simulink model "B_Inverter1"  (Simulink 8.4)
settings: Solver=ode45  StartTime=0.0  StopTime=1  RelTol=1e-3
libraries: powerlib x10
settings Model: Creator=ELECTRICAL-HOD  LastModifiedBy=INTEL

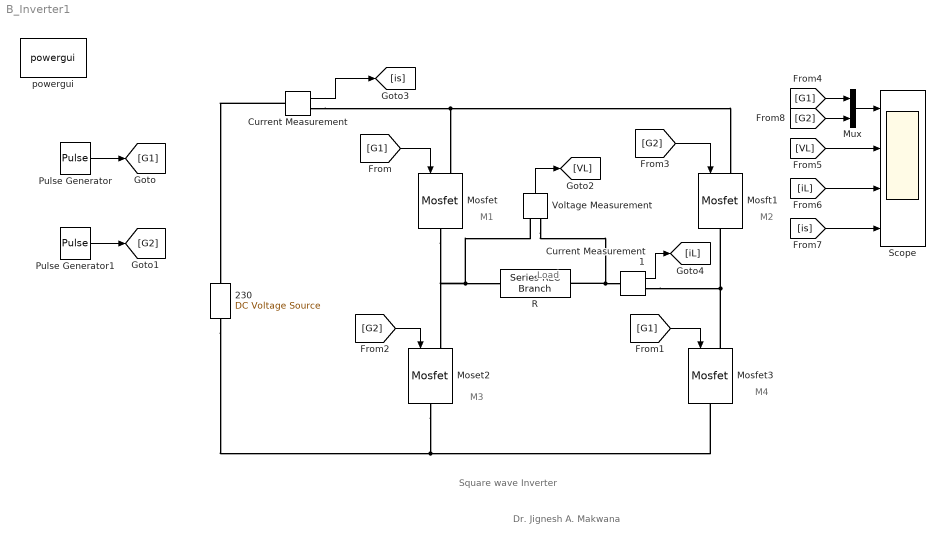
== system B_Inverter1 ==
  note: Load
  note: M1
  note: M4
  note: M3
  note: M2
  note: Dr. Jignesh A. Makwana
  note: Square wave Inverter
  230 : powerlib/Electrical Sources/DC Voltage Source  Amplitude=230  Measurements=None
  Current Measurement : powerlib/Measurements/Current Measurement  PhasorSimulation=off  OutputType=Complex  PSBequivalent=0
  Current Measurement1 : powerlib/Measurements/Current Measurement  PhasorSimulation=off  OutputType=Complex  PSBequivalent=0
  Moset2 : powerlib/Power Electronics/Mosfet  Ron=0.1  Lon=0  Rd=0.01  Vfd=0  IC=0  Rs=1e5  Cs=inf  Measurements=off
  Mosfet : powerlib/Power Electronics/Mosfet  Ron=0.1  Lon=0  Rd=0.01  Vfd=0  IC=0  Rs=1e5  Cs=inf  Measurements=off
  Mosfet3 : powerlib/Power Electronics/Mosfet  Ron=0.1  Lon=0  Rd=0.01  Vfd=0  IC=0  Rs=1e5  Cs=inf  Measurements=off
  Mosft1 : powerlib/Power Electronics/Mosfet  Ron=0.1  Lon=0  Rd=0.01  Vfd=0  IC=0  Rs=1e5  Cs=inf  Measurements=off
  Mux : Mux  Inputs=2
  Pulse Generator : DiscretePulseGenerator  PulseType=Time based  Amplitude=5  Period=0.02  PulseWidth=50
  Pulse Generator1 : DiscretePulseGenerator  PulseType=Time based  Amplitude=5  Period=0.02  PulseWidth=50  PhaseDelay=0.01
  R : powerlib/Elements/Series RLC Branch  LConnTagsString=__new0  RConnTagsString=__new0  BranchType=RL  Resistance=10  Inductance=10e-3  SetiL0=off  InitialCurrent=0  Capacitance=10e-6  Setx0=off  InitialVoltage=0  Measurements=None
  Scope : Scope  NumInputPorts=4
      settings: YMin=-5~-250~-25~-5  YMax=5~250~25~5
  Voltage Measurement : powerlib/Measurements/Voltage Measurement  PhasorSimulation=off  OutputType=Complex  PSBequivalent=0
  powergui : powerlib/powergui  Priority=1  SimulationMode=Continuous  SolverType=Tustin  SampleTime=50e-6  frequency=60  SPID=off  DisableSnubberDevices=off  DisableRonSwitches=off  DisableVfSwitches=off  SwTol=0  DisplayEquations=off  Interpol=off  methode=off  Ts=0  frequencyindice=0  Pbase=100e6  ErrMax=1e-4  Iterations=50  UnitsV=kV  UnitsW=MW  FunctionMessages=off  echomessages=off  HookPort=off  EnableUseOfTLC=off  x0status=blocks  RestoreLinks=warning  ResistiveCurrentMeasurement=off  Frange=[0:2:500]  Ylog=off  Xlog=on  ShowGrid=off  save=off  variable=ZData  structure=0  ZoomFFT=off  StartTime=0.0  cycles=1  DisplayStyle=1  fundamental=60  FreqAxis=off  MaxFrequency=1000  frequencyindicesteady=1  RmsSteady=1  display=off
  wires:
  Pulse Generator/1 -> [G1]
  [G1] -> Mosfet/1
  [G1] -> Mosfet3/1
  Pulse Generator1/1 -> [G2]
  [G2] -> Moset2/1
  [G2] -> Mosft1/1
  Voltage Measurement/1 -> [VL]
  Current Measurement/1 -> [is]
  Current Measurement1/1 -> [iL]
  [VL] -> Scope/2
  [iL] -> Scope/3
  [is] -> Scope/4
  Mux/1 -> Scope/1
  [G1] -> Mux/1
  [G2] -> Mux/2
  connections:
  Mosfet/RConn1 -- Moset2/LConn1 -- R/LConn1 -- Voltage Measurement/LConn1
  Voltage Measurement/LConn2 -- R/RConn1 -- Current Measurement1/LConn1
  230/LConn1 -- Mosfet3/RConn1 -- Moset2/RConn1
  Current Measurement/RConn1 -- Mosft1/LConn1 -- Mosfet/LConn1
  Current Measurement/LConn1 -- 230/RConn1
  Mosfet3/LConn1 -- Current Measurement1/RConn1 -- Mosft1/RConn1
